simulink model "thrust2omega"  (Simulink 8.7)
settings: Solver=VariableStepAuto  StartTime=0.0  StopTime=10.0  RelTol=1e-3
undefined symbols (not defined in the file): b, k, l
settings Model: Creator=mgreiff  LastModifiedBy=mgreiff
settings DataIOCC: LimitDataPoints=off  SaveFormat=Dataset
settings DebuggingCC: UnderspecifiedInitializationDetection=Simplified  MergeDetectMultiDrivingBlocksExec=error
settings HardwareCC: ProdBitPerPointer=64  ProdLargestAtomicFloat=Float  ProdIntDivRoundTo=Zero  ProdEndianess=LittleEndian  ProdWordSize=64  ProdHWDeviceType=Intel->x86-64 (Windows64)
settings ModelReferenceCC: PropagateSignalLabelsOutOfModel=on
settings ConfigComp: CovModelRefEnable=off

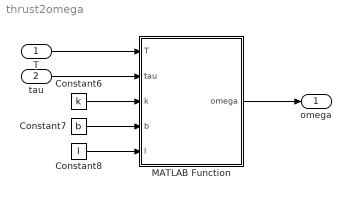
== system thrust2omega ==
  T : Inport  PortDimensions=1
  tau : Inport  Port=2  PortDimensions=3
  Constant6 : Constant  Value=k
  Constant7 : Constant  Value=b
  Constant8 : Constant  Value=l
  MATLAB Function : MATLAB Function  TreatAsAtomicUnit=on
  omega : Outport  PortDimensions=4
  wires:
  Constant7/1 -> MATLAB Function/4(b)
  tau/1 -> MATLAB Function/2(tau)
  Constant6/1 -> MATLAB Function/3(k)
  MATLAB Function/1(omega) -> omega/1
  T/1 -> MATLAB Function/1(T)
  Constant8/1 -> MATLAB Function/5(l)

== matlab function MATLAB Function ==
  data: T input double; omega output double; tau input double; k input double; b input double; l input double
function omega = Mw(T, tau, k, b, l)
%#codegen
tau_phi = tau(1);
tau_theta = tau(2);
tau_psi = tau(3);
w1sq = T/(4*k) - tau_theta/(2*k*l) - tau_psi / (4*b);
w2sq = T/(4*k) - tau_phi/(2*k*l) + tau_psi / (4*b);
w3sq = T/(4*k) + tau_theta/(2*k*l) - tau_psi / (4*b);
w4sq = T/(4*k) + tau_phi/(2*k*l) + tau_psi / (4*b);

omega = sqrt(max([w1sq w2sq w3sq w4sq]', 0));
